simulink model "model"  (R2014a)
(part 3 of 3)

  L_151069425/LConn3 -- T_151069425_150000_/RConn3 -- bus146/LConn1
  T_151077584_150000_/RConn1 -- L_151077584/LConn1
  T_151077584_150000_/RConn2 -- L_151077584/LConn2
  L_151077584/LConn3 -- T_151077584_150000_/RConn3 -- bus147/LConn1
  T_151109816__/RConn1 -- L_151109816/LConn1
  T_151109816__/RConn2 -- L_151109816/LConn2
  L_151109816/LConn3 -- T_151109816__/RConn3 -- bus148/LConn1
  T_151090496_150000;60000_Subestação_de_Ruivães/RConn1 -- L_151090496/LConn1
  T_151090496_150000;60000_Subestação_de_Ruivães/RConn2 -- L_151090496/LConn2
  L_151090496/LConn3 -- T_151090496_150000;60000_Subestação_de_Ruivães/RConn3 -- bus149/LConn1
  T_165898049_150000_/RConn1 -- L_165898049/LConn1
  T_165898049_150000_/RConn2 -- L_165898049/LConn2
  L_165898049/LConn3 -- T_165898049_150000_/RConn3 -- bus150/LConn1
  T_132614219_150000_/RConn1 -- L_132614219/LConn1
  T_132614219_150000_/RConn2 -- L_132614219/LConn2
  L_132614219/LConn3 -- T_132614219_150000_/RConn3 -- bus151/LConn1
  T_163226993_150000_Fogueteiro/RConn1 -- L_163226993/LConn1
  T_163226993_150000_Fogueteiro/RConn2 -- L_163226993/LConn2
  L_163226993/LConn3 -- T_163226993_150000_Fogueteiro/RConn3 -- bus152/LConn1
  T_151077580_150000_/RConn1 -- L_151077580/LConn1
  T_151077580_150000_/RConn2 -- L_151077580/LConn2
  L_151077580/LConn3 -- T_151077580_150000_/RConn3 -- bus153/LConn1
  T_151077578_150000;60000_/RConn1 -- L_151077578/LConn1
  T_151077578_150000;60000_/RConn2 -- L_151077578/LConn2
  L_151077578/LConn3 -- T_151077578_150000;60000_/RConn3 -- bus154/LConn1
  T_397005282__/RConn1 -- L_397005282/LConn1
  T_397005282__/RConn2 -- L_397005282/LConn2
  L_397005282/LConn3 -- T_397005282__/RConn3 -- bus155/LConn1
  T_151084399_150000_/RConn1 -- L_151084399/LConn1
  T_151084399_150000_/RConn2 -- L_151084399/LConn2
  L_151084399/LConn3 -- T_151084399_150000_/RConn3 -- bus156/LConn1
  T_163195990_150000_Subestação_de_Saboia/RConn1 -- L_163195990/LConn1
  T_163195990_150000_Subestação_de_Saboia/RConn2 -- L_163195990/LConn2
  L_163195990/LConn3 -- T_163195990_150000_Subestação_de_Saboia/RConn3 -- bus157/LConn1
  T_163195991_150000_Subestação_de_Luzianes/RConn1 -- L_163195991/LConn1
  T_163195991_150000_Subestação_de_Luzianes/RConn2 -- L_163195991/LConn2
  L_163195991/LConn3 -- T_163195991_150000_Subestação_de_Luzianes/RConn3 -- bus158/LConn1
  T_156176120_150000;60000_/RConn1 -- L_156176120/LConn1
  T_156176120_150000;60000_/RConn2 -- L_156176120/LConn2
  L_156176120/LConn3 -- T_156176120_150000;60000_/RConn3 -- bus159/LConn1
  T_144400130_220000_/RConn1 -- L_144400130/LConn1
  T_144400130_220000_/RConn2 -- L_144400130/LConn2
  L_144400130/LConn3 -- T_144400130_220000_/RConn3 -- bus160/LConn1
  T_144374439_220000_/RConn1 -- L_144374439/LConn1
  T_144374439_220000_/RConn2 -- L_144374439/LConn2
  L_144374439/LConn3 -- T_144374439_220000_/RConn3 -- bus161/LConn1
  T_144396420_220000;60000_Subestação_de_Régua/RConn1 -- L_144396420/LConn1
  T_144396420_220000;60000_Subestação_de_Régua/RConn2 -- L_144396420/LConn2
  L_144396420/LConn3 -- T_144396420_220000;60000_Subestação_de_Régua/RConn3 -- bus162/LConn1
  T_144398555_220000_Subestação_de_Vila_Pouca_de_Aguiar/RConn1 -- L_144398555/LConn1
  T_144398555_220000_Subestação_de_Vila_Pouca_de_Aguiar/RConn2 -- L_144398555/LConn2
  L_144398555/LConn3 -- T_144398555_220000_Subestação_de_Vila_Pouca_de_Aguiar/RConn3 -- bus163/LConn1
  T_126366408_220000;60000_Subestação_de_Urrô/RConn1 -- L_126366408/LConn1
  T_126366408_220000;60000_Subestação_de_Urrô/RConn2 -- L_126366408/LConn2
  L_126366408/LConn3 -- T_126366408_220000;60000_Subestação_de_Urrô/RConn3 -- bus164/LConn1
  T_127205502_220000_Subestação_de_Pocinho/RConn1 -- L_127205502/LConn1
  T_127205502_220000_Subestação_de_Pocinho/RConn2 -- L_127205502/LConn2
  L_127205502/LConn3 -- T_127205502_220000_Subestação_de_Pocinho/RConn3 -- bus165/LConn1
  T_144396428_220000_/RConn1 -- L_144396428/LConn1
  T_144396428_220000_/RConn2 -- L_144396428/LConn2
  L_144396428/LConn3 -- T_144396428_220000_/RConn3 -- bus166/LConn1
  T_127205641_220000_/RConn1 -- L_127205641/LConn1
  T_127205641_220000_/RConn2 -- L_127205641/LConn2
  L_127205641/LConn3 -- T_127205641_220000_/RConn3 -- bus167/LConn1
  T_151162379_150000;60000_Subestação_de_Mourisca/RConn1 -- L_151162379/LConn1
  T_151162379_150000;60000_Subestação_de_Mourisca/RConn2 -- L_151162379/LConn2
  L_151162379/LConn3 -- T_151162379_150000;60000_Subestação_de_Mourisca/RConn3 -- bus168/LConn1
  T_144545398_220000;60000_Subestação_de_Pereiros/RConn1 -- L_144545398/LConn1
  T_144545398_220000;60000_Subestação_de_Pereiros/RConn2 -- L_144545398/LConn2
  L_144545398/LConn3 -- T_144545398_220000;60000_Subestação_de_Pereiros/RConn3 -- bus169/LConn1
  T_144374442_220000;60000_Subestação_de_Estarreja/RConn1 -- L_144374442/LConn1
  T_144374442_220000;60000_Subestação_de_Estarreja/RConn2 -- L_144374442/LConn2
  L_144374442/LConn3 -- T_144374442_220000;60000_Subestação_de_Estarreja/RConn3 -- bus170/LConn1
  T_435865807__/RConn1 -- L_435865807/LConn1
  T_435865807__/RConn2 -- L_435865807/LConn2
  L_435865807/LConn3 -- T_435865807__/RConn3 -- bus171/LConn1
  T_24636062_220000_/RConn1 -- L_24636062/LConn1
  T_24636062_220000_/RConn2 -- L_24636062/LConn2
  L_24636062/LConn3 -- T_24636062_220000_/RConn3 -- bus172/LConn1
  T_144654759_220000_/RConn1 -- L_144654759/LConn1
  T_144654759_220000_/RConn2 -- L_144654759/LConn2
  L_144654759/LConn3 -- T_144654759_220000_/RConn3 -- bus173/LConn1
  T_144651478_220000_/RConn1 -- L_144651478/LConn1
  T_144651478_220000_/RConn2 -- L_144651478/LConn2
  L_144651478/LConn3 -- T_144651478_220000_/RConn3 -- bus174/LConn1
  T_151166980_220000_/RConn1 -- L_151166980/LConn1
  T_151166980_220000_/RConn2 -- L_151166980/LConn2
  L_151166980/LConn3 -- T_151166980_220000_/RConn3 -- bus175/LConn1
  T_144584585_220000;60000_Subestação_de_Tábua/RConn1 -- L_144584585/LConn1
  T_144584585_220000;60000_Subestação_de_Tábua/RConn2 -- L_144584585/LConn2
  L_144584585/LConn3 -- T_144584585_220000;60000_Subestação_de_Tábua/RConn3 -- bus176/LConn1
  T_144545399_220000_/RConn1 -- L_144545399/LConn1
  T_144545399_220000_/RConn2 -- L_144545399/LConn2
  L_144545399/LConn3 -- T_144545399_220000_/RConn3 -- bus177/LConn1
  T_144584580_220000_Subestação_de_Penela/RConn1 -- L_144584580/LConn1
  T_144584580_220000_Subestação_de_Penela/RConn2 -- L_144584580/LConn2
  L_144584580/LConn3 -- T_144584580_220000_Subestação_de_Penela/RConn3 -- bus178/LConn1
  T_144703168_220000_Subestação_de_Seixal/RConn1 -- L_144703168/LConn1
  T_144703168_220000_Subestação_de_Seixal/RConn2 -- L_144703168/LConn2
  L_144703168/LConn3 -- T_144703168_220000_Subestação_de_Seixal/RConn3 -- bus179/LConn1
  T_144596347_220000_Subestação_de_Santarém/RConn1 -- L_144596347/LConn1
  T_144596347_220000_Subestação_de_Santarém/RConn2 -- L_144596347/LConn2
  L_144596347/LConn3 -- T_144596347_220000_Subestação_de_Santarém/RConn3 -- bus180/LConn1
  T_151111218_220000_/RConn1 -- L_151111218/LConn1
  T_151111218_220000_/RConn2 -- L_151111218/LConn2
  L_151111218/LConn3 -- T_151111218_220000_/RConn3 -- bus181/LConn1
  T_144377301_220000;60000_Sub_Estação_de_Custóias/RConn1 -- L_144377301/LConn1
  T_144377301_220000;60000_Sub_Estação_de_Custóias/RConn2 -- L_144377301/LConn2
  L_144377301/LConn3 -- T_144377301_220000;60000_Sub_Estação_de_Custóias/RConn3 -- bus182/LConn1
  T_127205653_220000_/RConn1 -- L_127205653/LConn1
  T_127205653_220000_/RConn2 -- L_127205653/LConn2
  L_127205653/LConn3 -- T_127205653_220000_/RConn3 -- bus183/LConn1
  T_144387430_220000_/RConn1 -- L_144387430/LConn1
  T_144387430_220000_/RConn2 -- L_144387430/LConn2
  L_144387430/LConn3 -- T_144387430_220000_/RConn3 -- bus184/LConn1
  T_144385735_220000_/RConn1 -- L_144385735/LConn1
  T_144385735_220000_/RConn2 -- L_144385735/LConn2
  L_144385735/LConn3 -- T_144385735_220000_/RConn3 -- bus185/LConn1
  T_144588414_220000;60000_Subestação_REN_Zêzere/RConn1 -- L_144588414/LConn1
  T_144588414_220000;60000_Subestação_REN_Zêzere/RConn2 -- L_144588414/LConn2
  L_144588414/LConn3 -- T_144588414_220000;60000_Subestação_REN_Zêzere/RConn3 -- bus186/LConn1
  T_183668286_220000;60000_Subestação_de_Sete_Rios/RConn1 -- L_183668286/LConn1
  T_183668286_220000;60000_Subestação_de_Sete_Rios/RConn2 -- L_183668286/LConn2
  L_183668286/LConn3 -- T_183668286_220000;60000_Subestação_de_Sete_Rios/RConn3 -- bus187/LConn1
  T_144586949_220000_/RConn1 -- L_144586949/LConn1
  T_144586949_220000_/RConn2 -- L_144586949/LConn2
  L_144586949/LConn3 -- T_144586949_220000_/RConn3 -- bus188/LConn1
  T_142658477_220000_/RConn1 -- L_142658477/LConn1
  T_142658477_220000_/RConn2 -- L_142658477/LConn2
  L_142658477/LConn3 -- T_142658477_220000_/RConn3 -- bus189/LConn1
  T_116944631_220000;60000_Subestação_de_Canelas/RConn1 -- L_116944631/LConn1
  T_116944631_220000;60000_Subestação_de_Canelas/RConn2 -- L_116944631/LConn2
  L_116944631/LConn3 -- T_116944631_220000;60000_Subestação_de_Canelas/RConn3 -- bus190/LConn1
  T_47895778_220000_/RConn1 -- L_47895778/LConn1
  T_47895778_220000_/RConn2 -- L_47895778/LConn2
  L_47895778/LConn3 -- T_47895778_220000_/RConn3 -- bus191/LConn1
  T_137667702_220000;60000_Subestação_de_Vila_Chã/RConn1 -- L_137667702/LConn1
  T_137667702_220000;60000_Subestação_de_Vila_Chã/RConn2 -- L_137667702/LConn2
  L_137667702/LConn3 -- T_137667702_220000;60000_Subestação_de_Vila_Chã/RConn3 -- bus192/LConn1
  T_144552378_220000;150000;60000_/RConn1 -- L_144552378/LConn1
  T_144552378_220000;150000;60000_/RConn2 -- L_144552378/LConn2
  L_144552378/LConn3 -- T_144552378_220000;150000;60000_/RConn3 -- bus193/LConn1
  T_144432489_220000_Subestação_do_Ferro/RConn1 -- L_144432489/LConn1
  T_144432489_220000_Subestação_do_Ferro/RConn2 -- L_144432489/LConn2
  L_144432489/LConn3 -- T_144432489_220000_Subestação_do_Ferro/RConn3 -- bus194/LConn1
  T_144386243_220000_/RConn1 -- L_144386243/LConn1
  T_144386243_220000_/RConn2 -- L_144386243/LConn2
  L_144386243/LConn3 -- T_144386243_220000_/RConn3 -- bus195/LConn1
  T_144433994_220000_/RConn1 -- L_144433994/LConn1
  T_144433994_220000_/RConn2 -- L_144433994/LConn2
  L_144433994/LConn3 -- T_144433994_220000_/RConn3 -- bus196/LConn1
  T_144432478_220000_/RConn1 -- L_144432478/LConn1
  T_144432478_220000_/RConn2 -- L_144432478/LConn2
  L_144432478/LConn3 -- T_144432478_220000_/RConn3 -- bus197/LConn1
  T_144432485_220000_Subestação_de_Sobral/RConn1 -- L_144432485/LConn1
  T_144432485_220000_Subestação_de_Sobral/RConn2 -- L_144432485/LConn2
  L_144432485/LConn3 -- T_144432485_220000_Subestação_de_Sobral/RConn3 -- bus198/LConn1
  T_121159140_220000;60000_/RConn1 -- L_121159140/LConn1
  T_121159140_220000;60000_/RConn2 -- L_121159140/LConn2
  L_121159140/LConn3 -- T_121159140_220000;60000_/RConn3 -- bus199/LConn1
  T_144601080__/RConn1 -- L_144601080/LConn1
  T_144601080__/RConn2 -- L_144601080/LConn2
  L_144601080/LConn3 -- T_144601080__/RConn3 -- bus200/LConn1
  T_144608818_400000_/RConn1 -- L_144608818/LConn1
  T_144608818_400000_/RConn2 -- L_144608818/LConn2
  L_144608818/LConn3 -- T_144608818_400000_/RConn3 -- bus201/LConn1
  T_151162388_400000_/RConn1 -- L_151162388/LConn1
  T_151162388_400000_/RConn2 -- L_151162388/LConn2
  L_151162388/LConn3 -- T_151162388_400000_/RConn3 -- bus202/LConn1
  T_84526032_400000_/RConn1 -- L_84526032/LConn1
  T_84526032_400000_/RConn2 -- L_84526032/LConn2
  L_84526032/LConn3 -- T_84526032_400000_/RConn3 -- bus203/LConn1
  T_144573746_400000_/RConn1 -- L_144573746/LConn1
  T_144573746_400000_/RConn2 -- L_144573746/LConn2
  L_144573746/LConn3 -- T_144573746_400000_/RConn3 -- bus204/LConn1
  T_144554435_400000_Subestação_de_Lavos/RConn1 -- L_144554435/LConn1
  T_144554435_400000_Subestação_de_Lavos/RConn2 -- L_144554435/LConn2
  L_144554435/LConn3 -- T_144554435_400000_Subestação_de_Lavos/RConn3 -- bus205/LConn1
  T_144439472_220000_/RConn1 -- L_144439472/LConn1
  T_144439472_220000_/RConn2 -- L_144439472/LConn2
  L_144439472/LConn3 -- T_144439472_220000_/RConn3 -- bus206/LConn1
  T_144639174_400000;60000_Subestação_de_Alqueva/RConn1 -- L_144639174/LConn1
  T_144639174_400000;60000_Subestação_de_Alqueva/RConn2 -- L_144639174/LConn2
  L_144639174/LConn3 -- T_144639174_400000;60000_Subestação_de_Alqueva/RConn3 -- bus207/LConn1
  T_135457228_400000_/RConn1 -- L_135457228/LConn1
  T_135457228_400000_/RConn2 -- L_135457228/LConn2
  L_135457228/LConn3 -- T_135457228_400000_/RConn3 -- bus208/LConn1
  T_135457230_400000_/RConn1 -- L_135457230/LConn1
  T_135457230_400000_/RConn2 -- L_135457230/LConn2
  L_135457230/LConn3 -- T_135457230_400000_/RConn3 -- bus209/LConn1
  T_144708196_400000_/RConn1 -- L_144708196/LConn1
  T_144708196_400000_/RConn2 -- L_144708196/LConn2
  L_144708196/LConn3 -- T_144708196_400000_/RConn3 -- bus210/LConn1
  T_144327157_400000;220000_Subestación_de_Villarino/RConn1 -- L_144327157/LConn1
  T_144327157_400000;220000_Subestación_de_Villarino/RConn2 -- L_144327157/LConn2
  L_144327157/LConn3 -- T_144327157_400000;220000_Subestación_de_Villarino/RConn3 -- bus211/LConn1
